simulink model "ITACG_3D_salvo_simulation"  (R2023b)
settings: Solver=ode4  StartTime=0.0  StopTime=28  FixedStep=1/10  RelTol=1e-3
libraries: simulink_extras x40, simulink x4
(part 1 of 2)
settings Model: NumberOfSteps=10  PacingRate=5  Creator=Administrator  LastModifiedBy=Administrator
settings DebuggingCC: UnderSpecifiedDimensionMsg=warning

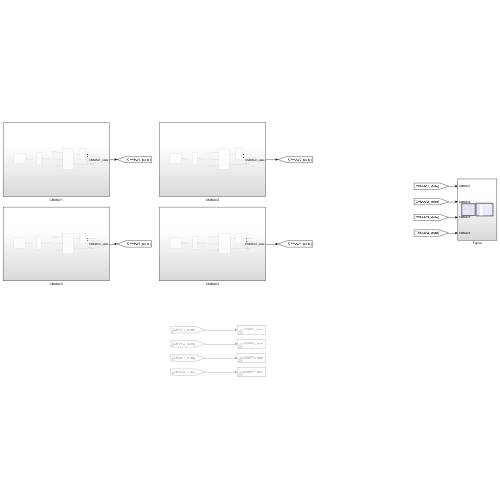
[thumbnail: Simulink's stored preview of the top-level diagram]
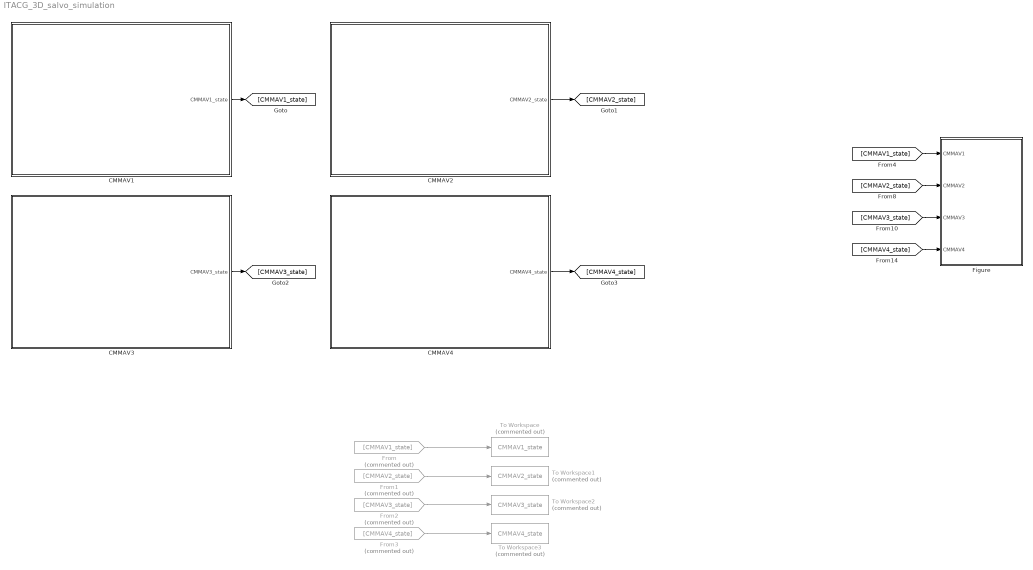
== system ITACG_3D_salvo_simulation ==
  CMMAV1 : Subsystem
  CMMAV2 : Subsystem
  CMMAV3 : Subsystem
  CMMAV4 : Subsystem
  Figure : Subsystem
  From : From  Commented=on  GotoTag=CMMAV1_state
  From1 : From  Commented=on  GotoTag=CMMAV2_state
  From2 : From  Commented=on  GotoTag=CMMAV3_state
  From3 : From  Commented=on  GotoTag=CMMAV4_state
  To Workspace : ToWorkspace  Commented=on  VariableName=CMMAV1_state  SaveFormat=Timeseries  SampleTime=-1
  To Workspace1 : ToWorkspace  Commented=on  VariableName=CMMAV2_state  SaveFormat=Timeseries  SampleTime=-1
  To Workspace2 : ToWorkspace  Commented=on  VariableName=CMMAV3_state  SaveFormat=Timeseries  SampleTime=-1
  To Workspace3 : ToWorkspace  Commented=on  VariableName=CMMAV4_state  SaveFormat=Timeseries  SampleTime=-1
  wires:
  CMMAV1/1(CMMAV1_state) -> [CMMAV1_state]
  CMMAV2/1(CMMAV2_state) -> [CMMAV2_state]
  CMMAV3/1(CMMAV3_state) -> [CMMAV3_state]
  CMMAV4/1(CMMAV4_state) -> [CMMAV4_state]
  From/1 -> To Workspace/1
  From1/1 -> To Workspace1/1
  From2/1 -> To Workspace2/1
  From3/1 -> To Workspace3/1
  [CMMAV2_state] -> Figure/2(CMMAV2)
  [CMMAV1_state] -> Figure/1(CMMAV1)
  [CMMAV3_state] -> Figure/3(CMMAV3)
  [CMMAV4_state] -> Figure/4(CMMAV4)

== system ITACG_3D_salvo_simulation/CMMAV1 ==
  Guidance : Subsystem
  Mux : Mux  Inputs=2
  Parameter init : Subsystem
  Point Mass Model : Subsystem
  Target : Subsystem  TreatAsAtomicUnit=on
  To File : ToFile  Filename=ITACG_CMMAV1.mat
  CMMAV1_state : Outport
  wires:
  [Parameter] -> Guidance/3(Parameter)
  [Taregt_info] -> Guidance/2(Target_info)
  [CMMAV1_state] -> Guidance/1(CMMAV1_state)
  Guidance/1(CMMAV1_input) -> Point Mass Model/1(CMMAV1_input)
  Parameter init/1(Parameter) -> [Parameter]
  Point Mass Model/1(CMMAV1_state) -> [CMMAV1_state], Mux/1, CMMAV1_state/1
  Target/1(Target_info) -> [Taregt_info]
  Mux/1 -> To File/1
  Guidance/2(sigma) -> Mux/2

== system ITACG_3D_salvo_simulation/CMMAV2 ==
  Guidance : Subsystem
  Mux : Mux  Inputs=2
  Parameter init : Subsystem
  Point Mass Model : Subsystem
  Target : Subsystem  TreatAsAtomicUnit=on
  To File : ToFile  Filename=ITACG_CMMAV2.mat
  CMMAV2_state : Outport
  wires:
  [Parameter] -> Guidance/3(Parameter)
  [Taregt_info] -> Guidance/2(Target_info)
  [CMMAV1_state] -> Guidance/1(CMMAV1_state)
  Guidance/1(CMMAV1_input) -> Point Mass Model/1(CMMAV1_input)
  Parameter init/1(Parameter) -> [Parameter]
  Target/1(Target_info) -> [Taregt_info]
  Point Mass Model/1(CMMAV1_state) -> CMMAV2_state/1, [CMMAV1_state], Mux/1
  Guidance/2(sigma) -> Mux/2
  Mux/1 -> To File/1

== system ITACG_3D_salvo_simulation/CMMAV3 ==
  Guidance : Subsystem
  Mux : Mux  Inputs=2
  Parameter init : Subsystem
  Point Mass Model : Subsystem
  Target : Subsystem  TreatAsAtomicUnit=on
  To File : ToFile  Filename=ITACG_CMMAV3.mat
  CMMAV3_state : Outport
  wires:
  [Parameter] -> Guidance/3(Parameter)
  [Taregt_info] -> Guidance/2(Target_info)
  [CMMAV1_state] -> Guidance/1(CMMAV1_state)
  Guidance/1(CMMAV1_input) -> Point Mass Model/1(CMMAV1_input)
  Parameter init/1(Parameter) -> [Parameter]
  Target/1(Target_info) -> [Taregt_info]
  Point Mass Model/1(CMMAV1_state) -> Mux/1, [CMMAV1_state], CMMAV3_state/1
  Guidance/2(sigma) -> Mux/2
  Mux/1 -> To File/1

== system ITACG_3D_salvo_simulation/CMMAV4 ==
  Guidance : Subsystem
  Mux : Mux  Inputs=2
  Parameter init : Subsystem
  Point Mass Model : Subsystem
  Target : Subsystem  TreatAsAtomicUnit=on
  To File : ToFile  Filename=ITACG_CMMAV4.mat
  CMMAV4_state : Outport
  wires:
  [Parameter] -> Guidance/3(Parameter)
  [Taregt_info] -> Guidance/2(Target_info)
  [CMMAV1_state] -> Guidance/1(CMMAV1_state)
  Guidance/1(CMMAV1_input) -> Point Mass Model/1(CMMAV1_input)
  Parameter init/1(Parameter) -> [Parameter]
  Target/1(Target_info) -> [Taregt_info]
  Point Mass Model/1(CMMAV1_state) -> Mux/1, [CMMAV1_state], CMMAV4_state/1
  Guidance/2(sigma) -> Mux/2
  Mux/1 -> To File/1

== system ITACG_3D_salvo_simulation/Figure ==
  note: Figure
  note: Input parameter
  CMMAV1 : Inport
  CMMAV2 : Inport  Port=2
  CMMAV3 : Inport  Port=3
  CMMAV4 : Inport  Port=4
  Bus Selector{,1..3} (4 alike) : BusSelector  OutputSignals=Pos_M_m
  Demux{,1..3} (4 alike) : Demux  Outputs=3
  MATLAB Function : MATLAB Function  TreatAsAtomicUnit=on
  wires:
  Demux/2 -> [CMMAV1_y]
  Demux/1 -> [CMMAV1_x]
  Demux/3 -> [CMMAV1_z]
  [CMMAV1] -> Demux/1
  CMMAV1/1 -> Bus Selector/1
  CMMAV2/1 -> Bus Selector1/1
  CMMAV3/1 -> Bus Selector2/1
  CMMAV4/1 -> Bus Selector3/1
  Bus Selector/1 -> [CMMAV1]  "<Pos_M_m>"
  Bus Selector1/1 -> [CMMAV2]  "<Pos_M_m>"
  Bus Selector2/1 -> [CMMAV3]  "<Pos_M_m>"
  Bus Selector3/1 -> [CMMAV4]  "<Pos_M_m>"
  Demux1/1 -> [CMMAV2_x]
  Demux1/3 -> [CMMAV2_z]
  Demux1/2 -> [CMMAV2_y]
  [CMMAV2] -> Demux1/1
  Demux2/2 -> [CMMAV3_y]
  Demux2/1 -> [CMMAV3_x]
  Demux2/3 -> [CMMAV3_z]
  [CMMAV3] -> Demux2/1
  Demux3/2 -> [CMMAV4_y]
  Demux3/1 -> [CMMAV4_x]
  Demux3/3 -> [CMMAV4_z]
  [CMMAV4] -> Demux3/1
  [CMMAV1_x] -> MATLAB Function/1(CMMAV1_x)
  [CMMAV1_y] -> MATLAB Function/2(CMMAV1_y)
  [CMMAV1_z] -> MATLAB Function/3(CMMAV1_z)
  [CMMAV2_x] -> MATLAB Function/4(CMMAV2_x)
  [CMMAV2_y] -> MATLAB Function/5(CMMAV2_y)
  [CMMAV2_z] -> MATLAB Function/6(CMMAV2_z)
  [CMMAV3_x] -> MATLAB Function/7(CMMAV3_x)
  [CMMAV3_y] -> MATLAB Function/8(CMMAV3_y)
  [CMMAV3_z] -> MATLAB Function/9(CMMAV3_z)
  [CMMAV4_x] -> MATLAB Function/10(CMMAV4_x)
  [CMMAV4_y] -> MATLAB Function/11(CMMAV4_y)
  [CMMAV4_z] -> MATLAB Function/12(CMMAV4_z)

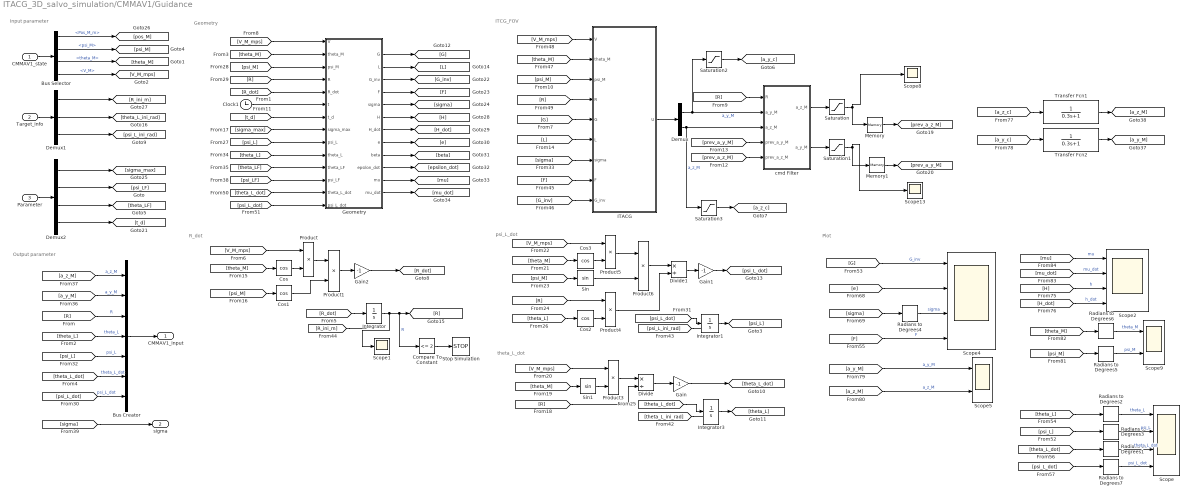
== system ITACG_3D_salvo_simulation/CMMAV1/Guidance ==
  note: Input parameter
  note: ITCG_FOV
  note: R_dot
  note: psi_L_dot
  note: theta_L_dot
  note: Output parameter
  note: Geometry
  note: Plot
  CMMAV1_state : Inport
  Target_info : Inport  Port=2
  Parameter : Inport  Port=3
  Bus Creator : BusCreator  Inputs=7
  Bus Selector : BusSelector  OutputSignals=Pos_M_m,psi_M,theta_M,V_M
  Clock1 : Clock
  Compare To Constant : simulink/Logic and Bit Operations/Compare To Constant  relop=<=  const=2  OutDataTypeStr=boolean
  Cos{,1..3} (4 alike) : Trigonometry  Operator=cos
  Demux : Demux  Outputs=2
  Demux1 : Demux  Outputs=3
  Demux2 : Demux
  Divide : Product  Inputs=*/
  Divide1 : Product  Inputs=*/
  Gain : Gain  Gain=-1
  Gain1 : Gain  Gain=-1
  Gain2 : Gain  Gain=-1
  Geometry : MATLAB Function  TreatAsAtomicUnit=on
  ITACG : MATLAB Function  TreatAsAtomicUnit=on
  Integrator : Integrator  InitialCondition=700
  Integrator1 : Integrator  InitialCondition=30*pi/180
  Integrator3 : Integrator  InitialCondition=-30*pi/180
  Memory : Memory
  Memory1 : Memory
  Product{,1,3..6} (6 alike) : Product
  Radians to Degrees{1..7} (7 alike) : simulink_extras/Transformations/Radians to Degrees
  Saturation{,1..3} (4 alike) : Saturate  UpperLimit=100  LowerLimit=-100
  Scope : Scope  NumInputPorts=4
  Scope1 : Scope
  Scope13 : Scope
  Scope2 : Scope  NumInputPorts=4
  Scope4 : Scope  NumInputPorts=4
  Scope5 : Scope  NumInputPorts=2
  Scope8 : Scope
  Scope9 : Scope  NumInputPorts=2
  Sin : Trigonometry
  Sin1 : Trigonometry
  Stop Simulation : Stop
  Transfer Fcn1 : TransferFcn  Denominator=[0.3 1]  ParameterTunability=Optimized
  Transfer Fcn2 : TransferFcn  Denominator=[0.3 1]  ParameterTunability=Optimized
  cmd Filter : MATLAB Function  TreatAsAtomicUnit=on
  CMMAV1_input : Outport
  sigma : Outport  Port=2
  wires:
  Product1/1 -> Gain2/1
  Gain2/1 -> [R_dot]
  [theta_L] -> Cos2/1
  [theta_L_dot] -> Integrator3/1
  Gain/1 -> [theta_L_dot]
  Product5/1 -> Product6/1
  Divide1/1 -> Gain1/1
  [V_M_mps] -> Product3/1
  [V_M_mps] -> Product5/1
  [theta_M] -> Sin1/1
  [R] -> Divide/2
  [theta_M] -> Cos3/1
  Divide/1 -> Gain/1
  [theta_M] -> Cos/1
  [R] -> Product4/1
  Product4/1 -> Divide1/2
  Integrator3/1 -> [theta_L]
  [psi_L_dot] -> Integrator1/1
  Sin1/1 -> Product3/2
  Product3/1 -> Divide/1
  [psi_M] -> Cos1/1
  Cos/1 -> Product/2
  Integrator1/1 -> [psi_L]
  Product6/1 -> Divide1/1
  [psi_M] -> Sin/1
  Compare To Constant/1 -> Stop Simulation/1
  [V_M_mps] -> Product/1
  Cos3/1 -> Product5/2
  Sin/1 -> Product6/2
  Integrator/1 -> Scope1/1, [R], Compare To Constant/1  "R"
  Product/1 -> Product1/1
  Cos2/1 -> Product4/2
  Cos1/1 -> Product1/2
  Gain1/1 -> [psi_L_dot]
  [R_dot] -> Integrator/1
  CMMAV1_state/1 -> Bus Selector/1
  Target_info/1 -> Demux1/1
  Demux2/1 -> [sigma_max]
  Parameter/1 -> Demux2/1
  Bus Selector/1 -> [pos_M]  "<Pos_M_m>"
  Bus Selector/4 -> [V_M_mps]  "<V_M>"
  Demux1/2 -> [theta_L_ini_rad]
  Demux1/3 -> [psi_L_ini_rad]
  Demux1/1 -> [R_ini_m]
  [psi_L] -> Bus Creator/5  "psi_L"
  [theta_L] -> Bus Creator/4  "theta_L"
  Bus Creator/1 -> CMMAV1_input/1
  [a_y_M] -> Bus Creator/2  "a_y_M"
  [R] -> Bus Creator/3  "R"
  [a_z_M] -> Bus Creator/1  "a_z_M"
  [theta_L_ini_rad] -> ?
  [psi_L_ini_rad] -> ?
  [R_ini_m] -> ?
  Bus Selector/2 -> [psi_M]  "<psi_M>"
  Bus Selector/3 -> [theta_M]  "<theta_M>"
  [psi_M] -> Geometry/3(psi_M)
  [V_M_mps] -> Geometry/1(V)
  [theta_M] -> Geometry/2(theta_M)
  [R] -> Geometry/4(R)
  Demux2/2 -> [psi_LF]
  Demux2/3 -> [theta_LF]
  Demux2/4 -> [t_d]
  Saturation2/1 -> [a_y_c]
  Saturation3/1 -> [a_z_c]
  cmd Filter/1(a_z_M) -> Saturation/1
  Memory/1 -> [prev_a_z_M]
  Transfer Fcn2/1 -> [a_y_M]
  Transfer Fcn1/1 -> [a_z_M]
  cmd Filter/2(a_y_M) -> Saturation1/1
  Saturation1/1 -> Scope13/1, Memory1/1
  Saturation/1 -> Scope8/1, Memory/1
  Demux/2 -> cmd Filter/3("a_z_M "), Saturation3/1  "a_z_M"
  [prev_a_y_M] -> cmd Filter/4(prev_a_y_M)
  [prev_a_z_M] -> cmd Filter/5(prev_a_z_M)
  [a_z_c] -> Transfer Fcn1/1
  Demux/1 -> cmd Filter/2("a_y_M "), Saturation2/1  "a_y_M"
  Memory1/1 -> [prev_a_y_M]
  [a_y_c] -> Transfer Fcn2/1
  [R] -> cmd Filter/1(R)
  ITACG/1(U) -> Demux/1
  [theta_LF] -> Geometry/11(theta_LF)
  [psi_LF] -> Geometry/12(psi_LF)
  [theta_L_dot] -> Geometry/13(theta_L_dot)
  [R_dot] -> Geometry/5(R_dot)
  [t_d] -> Geometry/7(t_d)
  [sigma_max] -> Geometry/8(sigma_max)
  [psi_L] -> Geometry/9(psi_L)
  [theta_L] -> Geometry/10(theta_L)
  [psi_L_dot] -> Geometry/14(psi_L_dot)
  Clock1/1 -> Geometry/6(t)
  Geometry/1(G) -> [G]
  Geometry/2(L) -> [L]
  Geometry/3(G_inv) -> [G_inv]
  Geometry/4(F) -> [F]
  Geometry/5(sigma) -> [sigma]
  Geometry/6(H) -> [H]
  Geometry/7(H_dot) -> [H_dot]
  Geometry/8(e) -> [e]
  Geometry/9(beta) -> [beta]
  Geometry/10(epsilon_dot) -> [epsilon_dot]
  Geometry/11(mu) -> [mu]
  Geometry/12(mu_dot) -> [mu_dot]
  [V_M_mps] -> ITACG/1(V)
  [theta_M] -> ITACG/2(theta_M)
  [psi_M] -> ITACG/3(psi_M)
  [G] -> ITACG/5(G)
  [L] -> ITACG/6(L)
  [sigma] -> ITACG/7(sigma)
  [F] -> ITACG/8(F)
  [G_inv] -> ITACG/9(G_inv)
  [R] -> ITACG/4(R)
  Radians to Degrees6/1 -> Scope9/1  "theta_M"
  Radians to Degrees7/1 -> Scope/4  "psi_L_dot"
  [psi_M] -> Radians to Degrees5/1
  [theta_L_dot] -> Radians to Degrees1/1
  Radians to Degrees3/1 -> Scope/2  "psi_L"
  [theta_L] -> Radians to Degrees2/1
  Radians to Degrees4/1 -> Scope4/3  "sigma"
  Radians to Degrees2/1 -> Scope/1  "theta_L"
  Radians to Degrees5/1 -> Scope9/2  "psi_M"
  [H] -> Scope2/3  "h"
  [psi_L] -> Radians to Degrees3/1
  [mu] -> Scope2/1  "mu"
  [mu_dot] -> Scope2/2  "mu_dot"
  Radians to Degrees1/1 -> Scope/3  "theta_L_dot"
  [sigma] -> Radians to Degrees4/1
  [a_y_M] -> Scope5/1  "a_y_M"
  [a_z_M] -> Scope5/2  "a_z_M"
  [G] -> Scope4/1  "G_inv"
  [theta_M] -> Radians to Degrees6/1
  [psi_L_dot] -> Radians to Degrees7/1
  [F] -> Scope4/4  "F"
  [H_dot] -> Scope2/4  "h_dot"
  [e] -> Scope4/2
  [theta_L_dot] -> Bus Creator/6  "theta_L_dot"
  [psi_L_dot] -> Bus Creator/7  "psi_L_dot"
  [sigma] -> sigma/1

== system ITACG_3D_salvo_simulation/CMMAV1/Parameter init ==
  Constant : Constant  Value=45
  Constant1 : Constant  Value=0
  Constant2 : Constant  Value=-60
  Constant3 : Constant  Value=28
  Degrees to Radians : simulink_extras/Transformations/Degrees to Radians
  Degrees to Radians1 : simulink_extras/Transformations/Degrees to Radians
  Degrees to Radians2 : simulink_extras/Transformations/Degrees to Radians
  Mux : Mux
  Parameter : Outport
  wires:
  Mux/1 -> Parameter/1
  Constant3/1 -> Mux/4  "t_d"
  Constant2/1 -> Degrees to Radians2/1
  Constant1/1 -> Degrees to Radians1/1
  Constant/1 -> Degrees to Radians/1
  Degrees to Radians2/1 -> Mux/3  "theta_LF"
  Degrees to Radians1/1 -> Mux/2  "psi_LF"
  Degrees to Radians/1 -> Mux/1  "sigma_max"

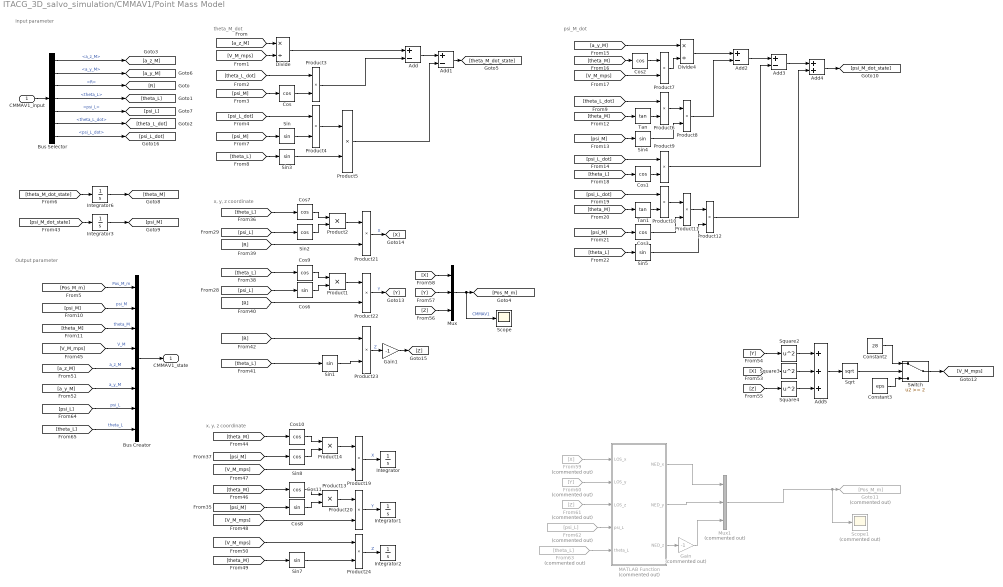
== system ITACG_3D_salvo_simulation/CMMAV1/Point Mass Model ==
  note: Input parameter
  note: x, y, z coordinate
  note: Output parameter
  note: x, y, z coordinate
  note: theta_M_dot
  note: psi_M_dot
  CMMAV1_input : Inport
  Add{,1..3} (4 alike) : Sum  Inputs=+-
  Add4 : Sum
  Add5 : Sum  Inputs=+++
  Bus Creator : BusCreator  Inputs=8
  Bus Selector : BusSelector  OutputSignals=a_z_M,a_y_M,R,theta_L,psi_L,theta_L_dot,psi_L_dot
  Constant2 : Constant  Value=28
  Constant3 : Constant  Value=eps
  Cos{,1..3,7,9..11} (8 alike) : Trigonometry  Operator=cos
  Cos6 : Trigonometry
  Cos8 : Trigonometry
  Divide : Product  Inputs=*/
  Divide4 : Product  Inputs=*/
  From59 : From  Commented=on  GotoTag=X
  From60 : From  Commented=on  GotoTag=Y
  From61 : From  Commented=on  GotoTag=Z
  From62 : From  Commented=on  GotoTag=psi_L
  From63 : From  Commented=on  GotoTag=theta_L
  Gain : Gain  Commented=on  Gain=-1
  Gain1 : Gain  Gain=-1
  Goto11 : Goto  Commented=on  GotoTag=Pos_M_m
  Integrator : Integrator
  Integrator1 : Integrator
  Integrator2 : Integrator
  Integrator3 : Integrator  InitialCondition=10*pi/180
  Integrator6 : Integrator  InitialCondition=10*pi/180
  MATLAB Function : MATLAB Function  Commented=on  TreatAsAtomicUnit=on
  Mux : Mux  Inputs=3
  Mux1 : Mux  Commented=on  Inputs=3
  Product{1..14,19..24} (20 alike) : Product
  Scope : Scope
  Scope1 : Scope  Commented=on
  Sin{,1,3..5,7} (6 alike) : Trigonometry
  Sin2 : Trigonometry  Operator=cos
  Sin8 : Trigonometry  Operator=cos
  Sqrt : Sqrt
  Square2 : Math  Operator=square
  Square3 : Math  Operator=square
  Square4 : Math  Operator=square
  Switch : Switch  Threshold=2  SaturateOnIntegerOverflow=off  InputSameDT=off
  Tan : Trigonometry  Operator=tan
  Tan1 : Trigonometry  Operator=tan
  CMMAV1_state : Outport
  wires:
  [psi_M] -> Bus Creator/2  "psi_M"
  [psi_M_dot_state] -> Integrator3/1
  [theta_L] -> Cos9/1
  [V_M_mps] -> Bus Creator/4  "V_M"
  Cos6/1 -> Product1/2
  Bus Selector/2 -> [a_y_M]  "<a_y_M>"
  Integrator6/1 -> [theta_M]
  [psi_L] -> Cos6/1
  Bus Selector/5 -> [psi_L]  "<psi_L>"
  Product21/1 -> [X]  "X"
  Product1/1 -> Product22/1
  Integrator3/1 -> [psi_M]
  Sin2/1 -> Product2/2
  Bus Selector/1 -> [a_z_M]  "<a_z_M>"
  Mux/1 -> [Pos_M_m], Scope/1  "CMMAV1"
  Bus Selector/3 -> [R]  "<R>"
  [theta_M] -> Bus Creator/3  "theta_M"
  [psi_L] -> Sin2/1
  Product2/1 -> Product21/1
  Cos9/1 -> Product1/1
  [theta_L] -> Cos7/1
  Cos7/1 -> Product2/1
  [theta_M_dot_state] -> Integrator6/1
  Product22/1 -> [Y]  "Y"
  [V_M_mps] -> Product24/1
  Sin7/1 -> Product24/2
  [V_M_mps] -> Product20/2
  [theta_M] -> Cos11/1
  [psi_M] -> Sin8/1
  [theta_M] -> Sin7/1
  Sin8/1 -> Product14/2
  Product14/1 -> Product19/1
  Product19/1 -> Integrator/1  "X"
  Product13/1 -> Product20/1
  Product24/1 -> Integrator2/1  "Z"
  [psi_M] -> Cos8/1
  [V_M_mps] -> Product19/2
  [theta_M] -> Cos10/1
  Cos11/1 -> Product13/1
  Cos8/1 -> Product13/2
  Product20/1 -> Integrator1/1  "Y"
  Cos10/1 -> Product14/1
  [R] -> Product21/2
  [R] -> Product22/2
  [R] -> Product23/1
  Sin1/1 -> Product23/2
  [theta_L] -> Sin1/1
  CMMAV1_input/1 -> Bus Selector/1
  [Pos_M_m] -> Bus Creator/1  "Pos_M_m"
  Bus Creator/1 -> CMMAV1_state/1
  Bus Selector/4 -> [theta_L]  "<theta_L>"
  [a_z_M] -> Bus Creator/5  "a_z_M"
  [a_y_M] -> Bus Creator/6  "a_y_M"
  Constant3/1 -> Switch/3
  Switch/1 -> [V_M_mps]
  Sqrt/1 -> Switch/2
  Add5/1 -> Sqrt/1
  Square2/1 -> Add5/1
  [Y] -> Square2/1
  Constant2/1 -> Switch/1
  [X] -> Square3/1
  Square3/1 -> Add5/2
  Product23/1 -> Gain1/1  "Z"
  [Z] -> Square4/1
  [X] -> Mux/1
  [Y] -> Mux/2
  [Z] -> Mux/3
  Square4/1 -> Add5/3
  From59/1 -> MATLAB Function/1(LOS_x)
  From60/1 -> MATLAB Function/2(LOS_y)
  From61/1 -> MATLAB Function/3(LOS_z)
  From62/1 -> MATLAB Function/4(psi_L)
  From63/1 -> MATLAB Function/5(theta_L)
  MATLAB Function/2(NED_y) -> Mux1/2
  MATLAB Function/1(NED_x) -> Mux1/1
  MATLAB Function/3(NED_z) -> Gain/1
  Gain/1 -> Mux1/3
  Mux1/1 -> Scope1/1, Goto11/1
  [psi_L] -> Bus Creator/7  "psi_L"
  [theta_L] -> Bus Creator/8  "theta_L"
  Product5/1 -> Add1/2
  Add/1 -> Add1/1
  Product4/1 -> Product5/1
  [a_z_M] -> Divide/1
  Divide/1 -> Add/1
  [V_M_mps] -> Divide/2
  Sin3/1 -> Product5/2
  Sin/1 -> Product4/2
  [psi_L_dot] -> Product4/1
  [psi_M] -> Cos/1
  Cos/1 -> Product3/2
  Add1/1 -> [theta_M_dot_state]
  Product3/1 -> Add/2
  [psi_M] -> Sin/1
  [theta_L] -> Sin3/1
  [theta_L_dot] -> Product3/1
  Product8/1 -> Add2/2
  [a_y_M] -> Divide4/1
  Product7/1 -> Divide4/2
  Divide4/1 -> Add2/1
  [V_M_mps] -> Product7/2
  Product6/1 -> Product8/1
  Product10/1 -> Product11/1
  Tan1/1 -> Product10/2
  [theta_L] -> Cos1/1
  Product12/1 -> Add4/2
  [theta_L] -> Sin5/1
  Product11/1 -> Product12/1
  [theta_L_dot] -> Product6/1
  Sin5/1 -> Product12/2
  Cos3/1 -> Product11/2
  [psi_M] -> Cos3/1
  Product9/1 -> Add3/2
  Add4/1 -> [psi_M_dot_state]
  [psi_L_dot] -> Product10/1
  [theta_M] -> Tan1/1
  Cos1/1 -> Product9/2
  [theta_M] -> Cos2/1
  Sin4/1 -> Product8/2
  [psi_M] -> Sin4/1
  [theta_M] -> Tan/1
  Tan/1 -> Product6/2
  [psi_L_dot] -> Product9/1
  Cos2/1 -> Product7/1
  Add2/1 -> Add3/1
  Add3/1 -> Add4/1
  Gain1/1 -> [Z]
  Bus Selector/6 -> [theta_L_dot]  "<theta_L_dot>"
  Bus Selector/7 -> [psi_L_dot]  "<psi_L_dot>"

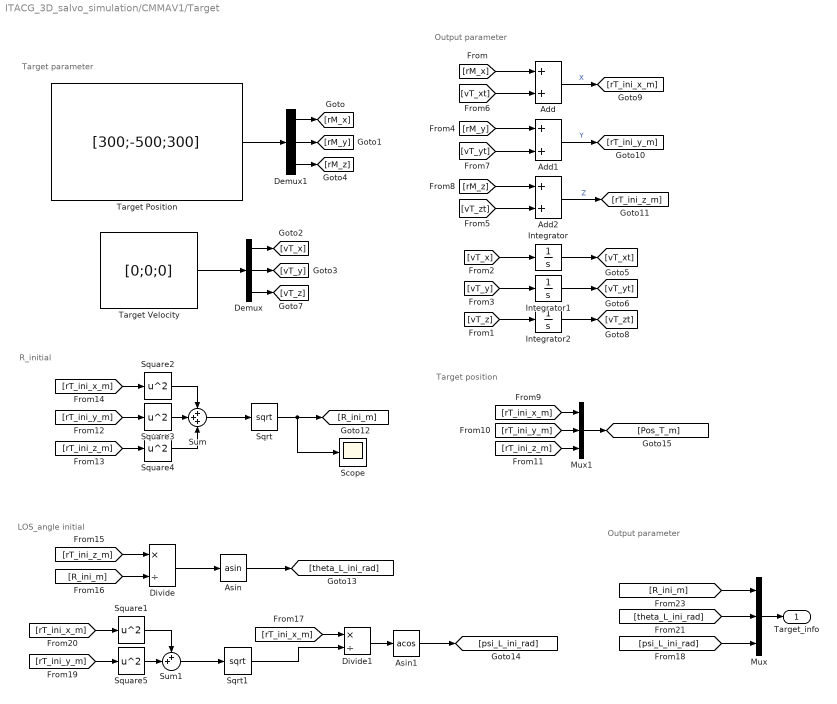
== system ITACG_3D_salvo_simulation/CMMAV1/Target ==
  note: LOS_angle initial
  note: Target position
  note: Target parameter
  note: Output parameter
  note: R_initial
  note: Output parameter
  Add : Sum
  Add1 : Sum
  Add2 : Sum
  Asin : Trigonometry  Operator=asin
  Asin1 : Trigonometry  Operator=acos
  Demux : Demux  Outputs=3
  Demux1 : Demux  Outputs=3
  Divide : Product  Inputs=*/
  Divide1 : Product  Inputs=*/
  Integrator : Integrator
  Integrator1 : Integrator
  Integrator2 : Integrator
  Mux : Mux  Inputs=3
  Mux1 : Mux  Inputs=3
  Scope : Scope
  Sqrt : Sqrt
  Sqrt1 : Sqrt
  Square{1..5} (5 alike) : Math  Operator=square
  Sum : Sum  Inputs=+++
  Sum1 : Sum  Inputs=++|
  Target Position : Constant  Value=[300;-500;300]  VectorParams1D=off
  Target Velocity : Constant  Value=[0;0;0]  VectorParams1D=off
  Target_info : Outport
  wires:
  [psi_L_ini_rad] -> Mux/3
  Asin/1 -> [theta_L_ini_rad]
  [rT_ini_z_m] -> Mux1/3
  [rM_z] -> Add2/1
  Demux/3 -> [vT_z]
  [vT_z] -> Integrator2/1
  Demux/2 -> [vT_y]
  [rT_ini_x_m] -> Mux1/1
  Add1/1 -> [rT_ini_y_m]  "Y"
  Square2/1 -> Sum/1
  [vT_x] -> Integrator/1
  Mux1/1 -> [Pos_T_m]
  Square3/1 -> Sum/2
  Add2/1 -> [rT_ini_z_m]  "Z"
  Integrator/1 -> [vT_xt]
  Sum/1 -> Sqrt/1
  Demux1/3 -> [rM_z]
  [rT_ini_y_m] -> Mux1/2
  Integrator1/1 -> [vT_yt]
  Demux/1 -> [vT_x]
  Demux1/1 -> [rM_x]
  Target Velocity/1 -> Demux/1
  Demux1/2 -> [rM_y]
  Add/1 -> [rT_ini_x_m]  "X"
  [vT_yt] -> Add1/2
  Divide1/1 -> Asin1/1
  [rM_x] -> Add/1
  [vT_zt] -> Add2/2
  Sum1/1 -> Sqrt1/1
  [rT_ini_x_m] -> Square1/1
  Square1/1 -> Sum1/1
  Square5/1 -> Sum1/2
  [rT_ini_y_m] -> Square5/1
  [vT_y] -> Integrator1/1
  [rM_y] -> Add1/1
  [rT_ini_z_m] -> Divide/1
  [R_ini_m] -> Mux/1
  Sqrt/1 -> Scope/1, [R_ini_m]
  [R_ini_m] -> Divide/2
  [rT_ini_z_m] -> Square4/1
  Sqrt1/1 -> Divide1/2
  [vT_xt] -> Add/2
  Divide/1 -> Asin/1
  Integrator2/1 -> [vT_zt]
  Square4/1 -> Sum/3
  [rT_ini_x_m] -> Divide1/1
  [theta_L_ini_rad] -> Mux/2
  Asin1/1 -> [psi_L_ini_rad]
  Mux/1 -> Target_info/1
  Target Position/1 -> Demux1/1
  [rT_ini_y_m] -> Square3/1
  [rT_ini_x_m] -> Square2/1

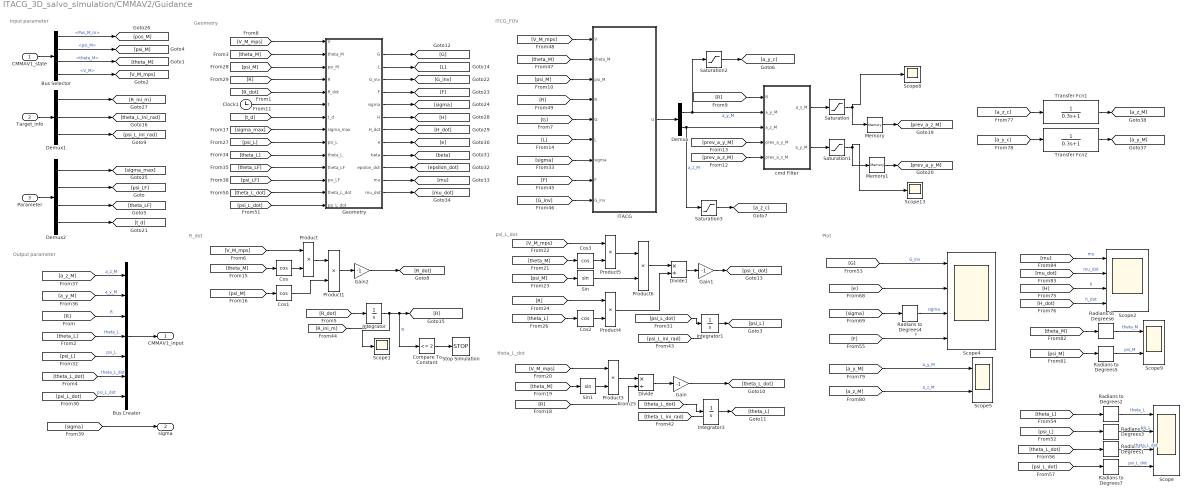
== system ITACG_3D_salvo_simulation/CMMAV2/Guidance ==
  note: Input parameter
  note: ITCG_FOV
  note: R_dot
  note: psi_L_dot
  note: theta_L_dot
  note: Output parameter
  note: Geometry
  note: Plot
  CMMAV1_state : Inport
  Target_info : Inport  Port=2
  Parameter : Inport  Port=3
  Bus Creator : BusCreator  Inputs=7
  Bus Selector : BusSelector  OutputSignals=Pos_M_m,psi_M,theta_M,V_M
  Clock1 : Clock
  Compare To Constant : simulink/Logic and Bit Operations/Compare To Constant  relop=<=  const=2  OutDataTypeStr=boolean
  Cos{,1..3} (4 alike) : Trigonometry  Operator=cos
  Demux : Demux  Outputs=2
  Demux1 : Demux  Outputs=3
  Demux2 : Demux
  Divide : Product  Inputs=*/
  Divide1 : Product  Inputs=*/
  Gain : Gain  Gain=-1
  Gain1 : Gain  Gain=-1
  Gain2 : Gain  Gain=-1
  Geometry : MATLAB Function  TreatAsAtomicUnit=on
  ITACG : MATLAB Function  TreatAsAtomicUnit=on
  Integrator : Integrator  InitialCondition=700
  Integrator1 : Integrator  InitialCondition=-30*pi/180
  Integrator3 : Integrator  InitialCondition=-30*pi/180
  Memory : Memory
  Memory1 : Memory
  Product{,1,3..6} (6 alike) : Product
  Radians to Degrees{1..7} (7 alike) : simulink_extras/Transformations/Radians to Degrees
  Saturation{,1..3} (4 alike) : Saturate  UpperLimit=100  LowerLimit=-100
  Scope : Scope  NumInputPorts=4
  Scope1 : Scope
  Scope13 : Scope
  Scope2 : Scope  NumInputPorts=4
  Scope4 : Scope  NumInputPorts=4
  Scope5 : Scope  NumInputPorts=2
  Scope8 : Scope
  Scope9 : Scope  NumInputPorts=2
  Sin : Trigonometry
  Sin1 : Trigonometry
  Stop Simulation : Stop
  Transfer Fcn1 : TransferFcn  Denominator=[0.3 1]  ParameterTunability=Optimized
  Transfer Fcn2 : TransferFcn  Denominator=[0.3 1]  ParameterTunability=Optimized
  cmd Filter : MATLAB Function  TreatAsAtomicUnit=on
  CMMAV1_input : Outport
  sigma : Outport  Port=2
  wires:
  Product1/1 -> Gain2/1
  Gain2/1 -> [R_dot]
  [theta_L] -> Cos2/1
  [theta_L_dot] -> Integrator3/1
  Gain/1 -> [theta_L_dot]
  Product5/1 -> Product6/1
  Divide1/1 -> Gain1/1
  [V_M_mps] -> Product3/1
  [V_M_mps] -> Product5/1
  [theta_M] -> Sin1/1
  [R] -> Divide/2
  [theta_M] -> Cos3/1
  Divide/1 -> Gain/1
  [theta_M] -> Cos/1
  [R] -> Product4/1
  Product4/1 -> Divide1/2
  Integrator3/1 -> [theta_L]
  [psi_L_dot] -> Integrator1/1
  Sin1/1 -> Product3/2
  Product3/1 -> Divide/1
  [psi_M] -> Cos1/1
  Cos/1 -> Product/2
  Integrator1/1 -> [psi_L]
  Product6/1 -> Divide1/1
  [psi_M] -> Sin/1
  Compare To Constant/1 -> Stop Simulation/1
  [V_M_mps] -> Product/1
  Cos3/1 -> Product5/2
  Sin/1 -> Product6/2
  Integrator/1 -> Scope1/1, [R], Compare To Constant/1  "R"
  Product/1 -> Product1/1
  Cos2/1 -> Product4/2
  Cos1/1 -> Product1/2
  Gain1/1 -> [psi_L_dot]
  [R_dot] -> Integrator/1
  CMMAV1_state/1 -> Bus Selector/1
  Target_info/1 -> Demux1/1
  Demux2/1 -> [sigma_max]
  Parameter/1 -> Demux2/1
  Bus Selector/1 -> [pos_M]  "<Pos_M_m>"
  Bus Selector/4 -> [V_M_mps]  "<V_M>"
  Demux1/2 -> [theta_L_ini_rad]
  Demux1/3 -> [psi_L_ini_rad]
  Demux1/1 -> [R_ini_m]
  [psi_L] -> Bus Creator/5  "psi_L"
  [theta_L] -> Bus Creator/4  "theta_L"
  Bus Creator/1 -> CMMAV1_input/1
  [a_y_M] -> Bus Creator/2  "a_y_M"
  [R] -> Bus Creator/3  "R"
  [a_z_M] -> Bus Creator/1  "a_z_M"
  [theta_L_ini_rad] -> ?
  [psi_L_ini_rad] -> ?
  [R_ini_m] -> ?
  Bus Selector/2 -> [psi_M]  "<psi_M>"
  Bus Selector/3 -> [theta_M]  "<theta_M>"
  [psi_M] -> Geometry/3(psi_M)
  [V_M_mps] -> Geometry/1(V)
  [theta_M] -> Geometry/2(theta_M)
  [R] -> Geometry/4(R)
  Demux2/2 -> [psi_LF]
  Demux2/3 -> [theta_LF]
  Demux2/4 -> [t_d]
  Saturation2/1 -> [a_y_c]
  Saturation3/1 -> [a_z_c]
  cmd Filter/1(a_z_M) -> Saturation/1
  Memory/1 -> [prev_a_z_M]
  Transfer Fcn2/1 -> [a_y_M]
  Transfer Fcn1/1 -> [a_z_M]
  cmd Filter/2(a_y_M) -> Saturation1/1
  Saturation1/1 -> Scope13/1, Memory1/1
  Saturation/1 -> Scope8/1, Memory/1
  Demux/2 -> cmd Filter/3("a_z_M "), Saturation3/1  "a_z_M"
  [prev_a_y_M] -> cmd Filter/4(prev_a_y_M)
  [prev_a_z_M] -> cmd Filter/5(prev_a_z_M)
  [a_z_c] -> Transfer Fcn1/1
  Demux/1 -> cmd Filter/2("a_y_M "), Saturation2/1  "a_y_M"
  Memory1/1 -> [prev_a_y_M]
  [a_y_c] -> Transfer Fcn2/1
  [R] -> cmd Filter/1(R)
  ITACG/1(U) -> Demux/1
  [theta_LF] -> Geometry/11(theta_LF)
  [psi_LF] -> Geometry/12(psi_LF)
  [theta_L_dot] -> Geometry/13(theta_L_dot)
  [R_dot] -> Geometry/5(R_dot)
  [t_d] -> Geometry/7(t_d)
  [sigma_max] -> Geometry/8(sigma_max)
  [psi_L] -> Geometry/9(psi_L)
  [theta_L] -> Geometry/10(theta_L)
  [psi_L_dot] -> Geometry/14(psi_L_dot)
  Clock1/1 -> Geometry/6(t)
  Geometry/1(G) -> [G]
  Geometry/2(L) -> [L]
  Geometry/3(G_inv) -> [G_inv]
  Geometry/4(F) -> [F]
  Geometry/5(sigma) -> [sigma]
  Geometry/6(H) -> [H]
  Geometry/7(H_dot) -> [H_dot]
  Geometry/8(e) -> [e]
  Geometry/9(beta) -> [beta]
  Geometry/10(epsilon_dot) -> [epsilon_dot]
  Geometry/11(mu) -> [mu]
  Geometry/12(mu_dot) -> [mu_dot]
  [V_M_mps] -> ITACG/1(V)
  [theta_M] -> ITACG/2(theta_M)
  [psi_M] -> ITACG/3(psi_M)
  [G] -> ITACG/5(G)
  [L] -> ITACG/6(L)
  [sigma] -> ITACG/7(sigma)
  [F] -> ITACG/8(F)
  [G_inv] -> ITACG/9(G_inv)
  [R] -> ITACG/4(R)
  Radians to Degrees6/1 -> Scope9/1  "theta_M"
  Radians to Degrees7/1 -> Scope/4  "psi_L_dot"
  [psi_M] -> Radians to Degrees5/1
  [theta_L_dot] -> Radians to Degrees1/1
  Radians to Degrees3/1 -> Scope/2  "psi_L"
  [theta_L] -> Radians to Degrees2/1
  Radians to Degrees4/1 -> Scope4/3  "sigma"
  Radians to Degrees2/1 -> Scope/1  "theta_L"
  Radians to Degrees5/1 -> Scope9/2  "psi_M"
  [H] -> Scope2/3  "h"
  [psi_L] -> Radians to Degrees3/1
  [mu] -> Scope2/1  "mu"
  [mu_dot] -> Scope2/2  "mu_dot"
  Radians to Degrees1/1 -> Scope/3  "theta_L_dot"
  [sigma] -> Radians to Degrees4/1
  [a_y_M] -> Scope5/1  "a_y_M"
  [a_z_M] -> Scope5/2  "a_z_M"
  [G] -> Scope4/1  "G_inv"
  [theta_M] -> Radians to Degrees6/1
  [psi_L_dot] -> Radians to Degrees7/1
  [F] -> Scope4/4  "F"
  [H_dot] -> Scope2/4  "h_dot"
  [e] -> Scope4/2
  [theta_L_dot] -> Bus Creator/6  "theta_L_dot"
  [psi_L_dot] -> Bus Creator/7  "psi_L_dot"
  [sigma] -> sigma/1

== system ITACG_3D_salvo_simulation/CMMAV2/Parameter init ==
  Constant : Constant  Value=45
  Constant1 : Constant  Value=0
  Constant2 : Constant  Value=-70
  Constant3 : Constant  Value=28
  Degrees to Radians : simulink_extras/Transformations/Degrees to Radians
  Degrees to Radians1 : simulink_extras/Transformations/Degrees to Radians
  Degrees to Radians2 : simulink_extras/Transformations/Degrees to Radians
  Mux : Mux
  Parameter : Outport
  wires:
  Mux/1 -> Parameter/1
  Constant3/1 -> Mux/4  "t_d"
  Constant2/1 -> Degrees to Radians2/1
  Constant1/1 -> Degrees to Radians1/1
  Constant/1 -> Degrees to Radians/1
  Degrees to Radians2/1 -> Mux/3  "theta_LF"
  Degrees to Radians1/1 -> Mux/2  "psi_LF"
  Degrees to Radians/1 -> Mux/1  "sigma_max"

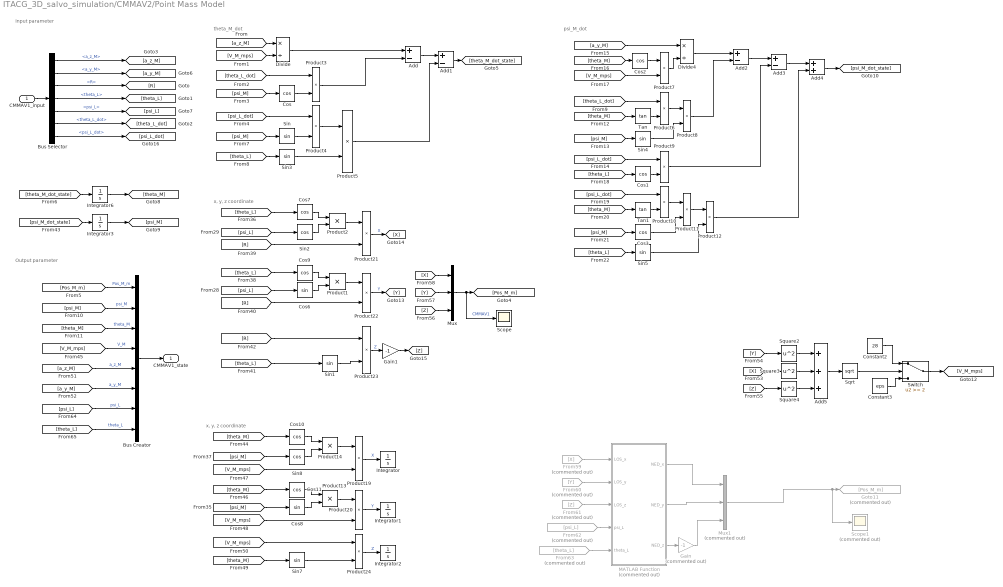
== system ITACG_3D_salvo_simulation/CMMAV2/Point Mass Model ==
  note: Input parameter
  note: x, y, z coordinate
  note: Output parameter
  note: x, y, z coordinate
  note: theta_M_dot
  note: psi_M_dot
  CMMAV1_input : Inport
  Add{,1..3} (4 alike) : Sum  Inputs=+-
  Add4 : Sum
  Add5 : Sum  Inputs=+++
  Bus Creator : BusCreator  Inputs=8
  Bus Selector : BusSelector  OutputSignals=a_z_M,a_y_M,R,theta_L,psi_L,theta_L_dot,psi_L_dot
  Constant2 : Constant  Value=28
  Constant3 : Constant  Value=eps
  Cos{,1..3,7,9..11} (8 alike) : Trigonometry  Operator=cos
  Cos6 : Trigonometry
  Cos8 : Trigonometry
  Divide : Product  Inputs=*/
  Divide4 : Product  Inputs=*/
  From59 : From  Commented=on  GotoTag=X
  From60 : From  Commented=on  GotoTag=Y
  From61 : From  Commented=on  GotoTag=Z
  From62 : From  Commented=on  GotoTag=psi_L
  From63 : From  Commented=on  GotoTag=theta_L
  Gain : Gain  Commented=on  Gain=-1
  Gain1 : Gain  Gain=-1
  Goto11 : Goto  Commented=on  GotoTag=Pos_M_m
  Integrator : Integrator
  Integrator1 : Integrator
  Integrator2 : Integrator
  Integrator3 : Integrator  InitialCondition=10*pi/180
  Integrator6 : Integrator  InitialCondition=10*pi/180
  MATLAB Function : MATLAB Function  Commented=on  TreatAsAtomicUnit=on
  Mux : Mux  Inputs=3
  Mux1 : Mux  Commented=on  Inputs=3
  Product{1..14,19..24} (20 alike) : Product
  Scope : Scope
  Scope1 : Scope  Commented=on
  Sin{,1,3..5,7} (6 alike) : Trigonometry
  Sin2 : Trigonometry  Operator=cos
  Sin8 : Trigonometry  Operator=cos
  Sqrt : Sqrt
  Square2 : Math  Operator=square
  Square3 : Math  Operator=square
  Square4 : Math  Operator=square
  Switch : Switch  Threshold=2  SaturateOnIntegerOverflow=off  InputSameDT=off
  Tan : Trigonometry  Operator=tan
  Tan1 : Trigonometry  Operator=tan
  CMMAV1_state : Outport
  wires:
  [psi_M] -> Bus Creator/2  "psi_M"
  [psi_M_dot_state] -> Integrator3/1
  [theta_L] -> Cos9/1
  [V_M_mps] -> Bus Creator/4  "V_M"
  Cos6/1 -> Product1/2
  Bus Selector/2 -> [a_y_M]  "<a_y_M>"
  Integrator6/1 -> [theta_M]
  [psi_L] -> Cos6/1
  Bus Selector/5 -> [psi_L]  "<psi_L>"
  Product21/1 -> [X]  "X"
  Product1/1 -> Product22/1
  Integrator3/1 -> [psi_M]
  Sin2/1 -> Product2/2
  Bus Selector/1 -> [a_z_M]  "<a_z_M>"
  Mux/1 -> [Pos_M_m], Scope/1  "CMMAV1"
  Bus Selector/3 -> [R]  "<R>"
  [theta_M] -> Bus Creator/3  "theta_M"
  [psi_L] -> Sin2/1
  Product2/1 -> Product21/1
  Cos9/1 -> Product1/1
  [theta_L] -> Cos7/1
  Cos7/1 -> Product2/1
  [theta_M_dot_state] -> Integrator6/1
  Product22/1 -> [Y]  "Y"
  [V_M_mps] -> Product24/1
  Sin7/1 -> Product24/2
  [V_M_mps] -> Product20/2
  [theta_M] -> Cos11/1
  [psi_M] -> Sin8/1
  [theta_M] -> Sin7/1
  Sin8/1 -> Product14/2
  Product14/1 -> Product19/1
  Product19/1 -> Integrator/1  "X"
  Product13/1 -> Product20/1
  Product24/1 -> Integrator2/1  "Z"
  [psi_M] -> Cos8/1
  [V_M_mps] -> Product19/2
  [theta_M] -> Cos10/1
  Cos11/1 -> Product13/1
  Cos8/1 -> Product13/2
  Product20/1 -> Integrator1/1  "Y"
  Cos10/1 -> Product14/1
  [R] -> Product21/2
  [R] -> Product22/2
  [R] -> Product23/1
  Sin1/1 -> Product23/2
  [theta_L] -> Sin1/1
  CMMAV1_input/1 -> Bus Selector/1
  [Pos_M_m] -> Bus Creator/1  "Pos_M_m"
  Bus Creator/1 -> CMMAV1_state/1
  Bus Selector/4 -> [theta_L]  "<theta_L>"
  [a_z_M] -> Bus Creator/5  "a_z_M"
  [a_y_M] -> Bus Creator/6  "a_y_M"
  Constant3/1 -> Switch/3
  Switch/1 -> [V_M_mps]
  Sqrt/1 -> Switch/2
  Add5/1 -> Sqrt/1
  Square2/1 -> Add5/1
  [Y] -> Square2/1
  Constant2/1 -> Switch/1
  [X] -> Square3/1
  Square3/1 -> Add5/2
  Product23/1 -> Gain1/1  "Z"
  [Z] -> Square4/1
  [X] -> Mux/1
  [Y] -> Mux/2
  [Z] -> Mux/3
  Square4/1 -> Add5/3
  From59/1 -> MATLAB Function/1(LOS_x)
  From60/1 -> MATLAB Function/2(LOS_y)
  From61/1 -> MATLAB Function/3(LOS_z)
  From62/1 -> MATLAB Function/4(psi_L)
  From63/1 -> MATLAB Function/5(theta_L)
  MATLAB Function/2(NED_y) -> Mux1/2
  MATLAB Function/1(NED_x) -> Mux1/1
  MATLAB Function/3(NED_z) -> Gain/1
  Gain/1 -> Mux1/3
  Mux1/1 -> Scope1/1, Goto11/1
  [psi_L] -> Bus Creator/7  "psi_L"
  [theta_L] -> Bus Creator/8  "theta_L"
  Product5/1 -> Add1/2
  Add/1 -> Add1/1
  Product4/1 -> Product5/1
  [a_z_M] -> Divide/1
  Divide/1 -> Add/1
  [V_M_mps] -> Divide/2
  Sin3/1 -> Product5/2
  Sin/1 -> Product4/2
  [psi_L_dot] -> Product4/1
  [psi_M] -> Cos/1
  Cos/1 -> Product3/2
  Add1/1 -> [theta_M_dot_state]
  Product3/1 -> Add/2
  [psi_M] -> Sin/1
  [theta_L] -> Sin3/1
  [theta_L_dot] -> Product3/1
  Product8/1 -> Add2/2
  [a_y_M] -> Divide4/1
  Product7/1 -> Divide4/2
  Divide4/1 -> Add2/1
  [V_M_mps] -> Product7/2
  Product6/1 -> Product8/1
  Product10/1 -> Product11/1
  Tan1/1 -> Product10/2
  [theta_L] -> Cos1/1
  Product12/1 -> Add4/2
  [theta_L] -> Sin5/1
  Product11/1 -> Product12/1
  [theta_L_dot] -> Product6/1
  Sin5/1 -> Product12/2
  Cos3/1 -> Product11/2
  [psi_M] -> Cos3/1
  Product9/1 -> Add3/2
  Add4/1 -> [psi_M_dot_state]
  [psi_L_dot] -> Product10/1
  [theta_M] -> Tan1/1
  Cos1/1 -> Product9/2
  [theta_M] -> Cos2/1
  Sin4/1 -> Product8/2
  [psi_M] -> Sin4/1
  [theta_M] -> Tan/1
  Tan/1 -> Product6/2
  [psi_L_dot] -> Product9/1
  Cos2/1 -> Product7/1
  Add2/1 -> Add3/1
  Add3/1 -> Add4/1
  Gain1/1 -> [Z]
  Bus Selector/6 -> [theta_L_dot]  "<theta_L_dot>"
  Bus Selector/7 -> [psi_L_dot]  "<psi_L_dot>"

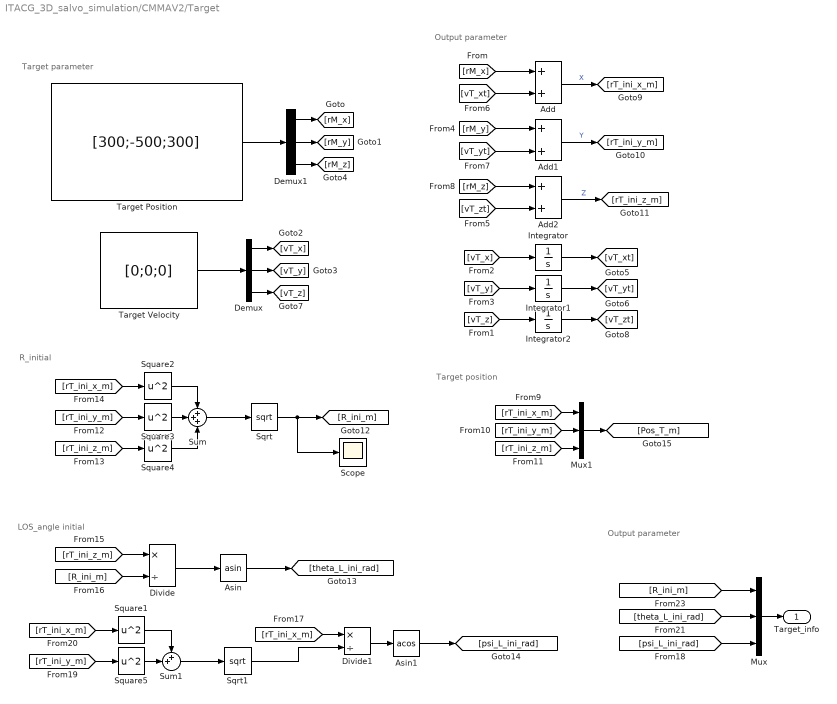
== system ITACG_3D_salvo_simulation/CMMAV2/Target ==
  note: LOS_angle initial
  note: Target position
  note: Target parameter
  note: Output parameter
  note: R_initial
  note: Output parameter
  Add : Sum
  Add1 : Sum
  Add2 : Sum
  Asin : Trigonometry  Operator=asin
  Asin1 : Trigonometry  Operator=acos
  Demux : Demux  Outputs=3
  Demux1 : Demux  Outputs=3
  Divide : Product  Inputs=*/
  Divide1 : Product  Inputs=*/
  Integrator : Integrator
  Integrator1 : Integrator
  Integrator2 : Integrator
  Mux : Mux  Inputs=3
  Mux1 : Mux  Inputs=3
  Scope : Scope
  Sqrt : Sqrt
  Sqrt1 : Sqrt
  Square{1..5} (5 alike) : Math  Operator=square
  Sum : Sum  Inputs=+++
  Sum1 : Sum  Inputs=++|
  Target Position : Constant  Value=[300;-500;300]  VectorParams1D=off
  Target Velocity : Constant  Value=[0;0;0]  VectorParams1D=off
  Target_info : Outport
  wires:
  [psi_L_ini_rad] -> Mux/3
  Asin/1 -> [theta_L_ini_rad]
  [rT_ini_z_m] -> Mux1/3
  [rM_z] -> Add2/1
  Demux/3 -> [vT_z]
  [vT_z] -> Integrator2/1
  Demux/2 -> [vT_y]
  [rT_ini_x_m] -> Mux1/1
  Add1/1 -> [rT_ini_y_m]  "Y"
  Square2/1 -> Sum/1
  [vT_x] -> Integrator/1
  Mux1/1 -> [Pos_T_m]
  Square3/1 -> Sum/2
  Add2/1 -> [rT_ini_z_m]  "Z"
  Integrator/1 -> [vT_xt]
  Sum/1 -> Sqrt/1
  Demux1/3 -> [rM_z]
  [rT_ini_y_m] -> Mux1/2
  Integrator1/1 -> [vT_yt]
  Demux/1 -> [vT_x]
  Demux1/1 -> [rM_x]
  Target Velocity/1 -> Demux/1
  Demux1/2 -> [rM_y]
  Add/1 -> [rT_ini_x_m]  "X"
  [vT_yt] -> Add1/2
  Divide1/1 -> Asin1/1
  [rM_x] -> Add/1
  [vT_zt] -> Add2/2
  Sum1/1 -> Sqrt1/1
  [rT_ini_x_m] -> Square1/1
  Square1/1 -> Sum1/1
  Square5/1 -> Sum1/2
  [rT_ini_y_m] -> Square5/1
  [vT_y] -> Integrator1/1
  [rM_y] -> Add1/1
  [rT_ini_z_m] -> Divide/1
  [R_ini_m] -> Mux/1
  Sqrt/1 -> Scope/1, [R_ini_m]
  [R_ini_m] -> Divide/2
  [rT_ini_z_m] -> Square4/1
  Sqrt1/1 -> Divide1/2
  [vT_xt] -> Add/2
  Divide/1 -> Asin/1
  Integrator2/1 -> [vT_zt]
  Square4/1 -> Sum/3
  [rT_ini_x_m] -> Divide1/1
  [theta_L_ini_rad] -> Mux/2
  Asin1/1 -> [psi_L_ini_rad]
  Mux/1 -> Target_info/1
  Target Position/1 -> Demux1/1
  [rT_ini_y_m] -> Square3/1
  [rT_ini_x_m] -> Square2/1

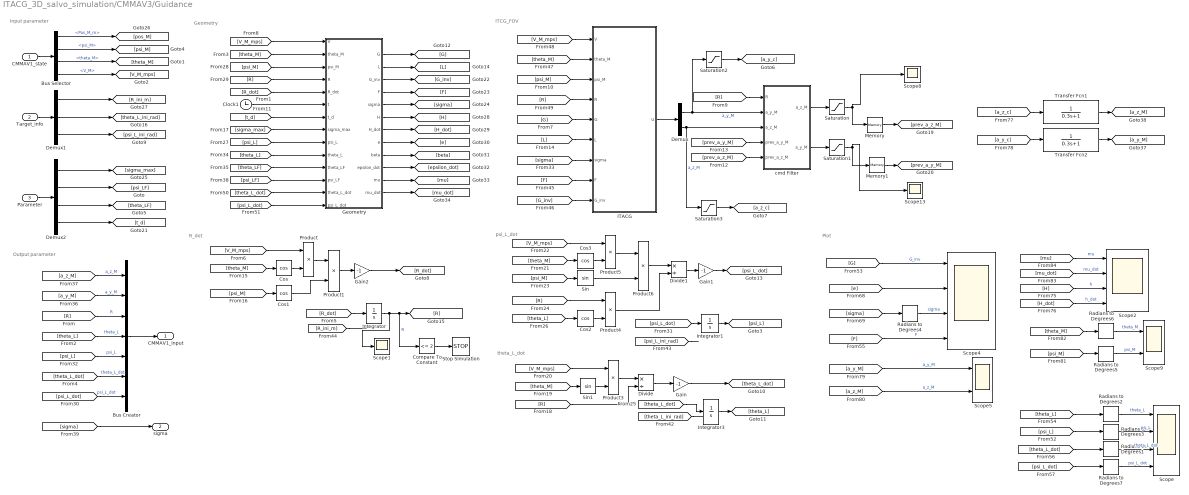
== system ITACG_3D_salvo_simulation/CMMAV3/Guidance ==
  note: Input parameter
  note: ITCG_FOV
  note: R_dot
  note: psi_L_dot
  note: theta_L_dot
  note: Output parameter
  note: Geometry
  note: Plot
  CMMAV1_state : Inport
  Target_info : Inport  Port=2
  Parameter : Inport  Port=3
  Bus Creator : BusCreator  Inputs=7
  Bus Selector : BusSelector  OutputSignals=Pos_M_m,psi_M,theta_M,V_M
  Clock1 : Clock
  Compare To Constant : simulink/Logic and Bit Operations/Compare To Constant  relop=<=  const=2  OutDataTypeStr=boolean
  Cos{,1..3} (4 alike) : Trigonometry  Operator=cos
  Demux : Demux  Outputs=2
  Demux1 : Demux  Outputs=3
  Demux2 : Demux
  Divide : Product  Inputs=*/
  Divide1 : Product  Inputs=*/
  Gain : Gain  Gain=-1
  Gain1 : Gain  Gain=-1
  Gain2 : Gain  Gain=-1
  Geometry : MATLAB Function  TreatAsAtomicUnit=on
  ITACG : MATLAB Function  TreatAsAtomicUnit=on
  Integrator : Integrator  InitialCondition=700
  Integrator1 : Integrator  InitialCondition=20*pi/180
  Integrator3 : Integrator  InitialCondition=-10*pi/180
  Memory : Memory
  Memory1 : Memory
  Product{,1,3..6} (6 alike) : Product
  Radians to Degrees{1..7} (7 alike) : simulink_extras/Transformations/Radians to Degrees
  Saturation{,1..3} (4 alike) : Saturate  UpperLimit=100  LowerLimit=-100
  Scope : Scope  NumInputPorts=4
  Scope1 : Scope
  Scope13 : Scope
  Scope2 : Scope  NumInputPorts=4
  Scope4 : Scope  NumInputPorts=4
  Scope5 : Scope  NumInputPorts=2
  Scope8 : Scope
  Scope9 : Scope  NumInputPorts=2
  Sin : Trigonometry
  Sin1 : Trigonometry
  Stop Simulation : Stop
  Transfer Fcn1 : TransferFcn  Denominator=[0.3 1]  ParameterTunability=Optimized
  Transfer Fcn2 : TransferFcn  Denominator=[0.3 1]  ParameterTunability=Optimized
  cmd Filter : MATLAB Function  TreatAsAtomicUnit=on
  CMMAV1_input : Outport
  sigma : Outport  Port=2
  wires:
  Product1/1 -> Gain2/1
  Gain2/1 -> [R_dot]
  [theta_L] -> Cos2/1
  [theta_L_dot] -> Integrator3/1
  Gain/1 -> [theta_L_dot]
  Product5/1 -> Product6/1
  Divide1/1 -> Gain1/1
  [V_M_mps] -> Product3/1
  [V_M_mps] -> Product5/1
  [theta_M] -> Sin1/1
  [R] -> Divide/2
  [theta_M] -> Cos3/1
  Divide/1 -> Gain/1
  [theta_M] -> Cos/1
  [R] -> Product4/1
  Product4/1 -> Divide1/2
  Integrator3/1 -> [theta_L]
  [psi_L_dot] -> Integrator1/1
  Sin1/1 -> Product3/2
  Product3/1 -> Divide/1
  [psi_M] -> Cos1/1
  Cos/1 -> Product/2
  Integrator1/1 -> [psi_L]
  Product6/1 -> Divide1/1
  [psi_M] -> Sin/1
  Compare To Constant/1 -> Stop Simulation/1
  [V_M_mps] -> Product/1
  Cos3/1 -> Product5/2
  Sin/1 -> Product6/2
  Integrator/1 -> Scope1/1, [R], Compare To Constant/1  "R"
  Product/1 -> Product1/1
  Cos2/1 -> Product4/2
  Cos1/1 -> Product1/2
  Gain1/1 -> [psi_L_dot]
  [R_dot] -> Integrator/1
  CMMAV1_state/1 -> Bus Selector/1
  Target_info/1 -> Demux1/1
  Demux2/1 -> [sigma_max]
  Parameter/1 -> Demux2/1
  Bus Selector/1 -> [pos_M]  "<Pos_M_m>"
  Bus Selector/4 -> [V_M_mps]  "<V_M>"
  Demux1/2 -> [theta_L_ini_rad]
  Demux1/3 -> [psi_L_ini_rad]
  Demux1/1 -> [R_ini_m]
  [psi_L] -> Bus Creator/5  "psi_L"
  [theta_L] -> Bus Creator/4  "theta_L"
  Bus Creator/1 -> CMMAV1_input/1
  [a_y_M] -> Bus Creator/2  "a_y_M"
  [R] -> Bus Creator/3  "R"
  [a_z_M] -> Bus Creator/1  "a_z_M"
  [theta_L_ini_rad] -> ?
  [psi_L_ini_rad] -> ?
  [R_ini_m] -> ?
  Bus Selector/2 -> [psi_M]  "<psi_M>"
  Bus Selector/3 -> [theta_M]  "<theta_M>"
  [psi_M] -> Geometry/3(psi_M)
  [V_M_mps] -> Geometry/1(V)
  [theta_M] -> Geometry/2(theta_M)
  [R] -> Geometry/4(R)
  Demux2/2 -> [psi_LF]
  Demux2/3 -> [theta_LF]
  Demux2/4 -> [t_d]
  Saturation2/1 -> [a_y_c]
  Saturation3/1 -> [a_z_c]
  cmd Filter/1(a_z_M) -> Saturation/1
  Memory/1 -> [prev_a_z_M]
  Transfer Fcn2/1 -> [a_y_M]
  Transfer Fcn1/1 -> [a_z_M]
  cmd Filter/2(a_y_M) -> Saturation1/1
  Saturation1/1 -> Scope13/1, Memory1/1
  Saturation/1 -> Scope8/1, Memory/1
  Demux/2 -> cmd Filter/3("a_z_M "), Saturation3/1  "a_z_M"
  [prev_a_y_M] -> cmd Filter/4(prev_a_y_M)
  [prev_a_z_M] -> cmd Filter/5(prev_a_z_M)
  [a_z_c] -> Transfer Fcn1/1
  Demux/1 -> cmd Filter/2("a_y_M "), Saturation2/1  "a_y_M"
  Memory1/1 -> [prev_a_y_M]
  [a_y_c] -> Transfer Fcn2/1
  [R] -> cmd Filter/1(R)
  ITACG/1(U) -> Demux/1
  [theta_LF] -> Geometry/11(theta_LF)
  [psi_LF] -> Geometry/12(psi_LF)
  [theta_L_dot] -> Geometry/13(theta_L_dot)
  [R_dot] -> Geometry/5(R_dot)
  [t_d] -> Geometry/7(t_d)
  [sigma_max] -> Geometry/8(sigma_max)
  [psi_L] -> Geometry/9(psi_L)
  [theta_L] -> Geometry/10(theta_L)
  [psi_L_dot] -> Geometry/14(psi_L_dot)
  Clock1/1 -> Geometry/6(t)
  Geometry/1(G) -> [G]
  Geometry/2(L) -> [L]
  Geometry/3(G_inv) -> [G_inv]
  Geometry/4(F) -> [F]
  Geometry/5(sigma) -> [sigma]
  Geometry/6(H) -> [H]
  Geometry/7(H_dot) -> [H_dot]
  Geometry/8(e) -> [e]
  Geometry/9(beta) -> [beta]
  Geometry/10(epsilon_dot) -> [epsilon_dot]
  Geometry/11(mu) -> [mu]
  Geometry/12(mu_dot) -> [mu_dot]
  [V_M_mps] -> ITACG/1(V)
  [theta_M] -> ITACG/2(theta_M)
  [psi_M] -> ITACG/3(psi_M)
  [G] -> ITACG/5(G)
  [L] -> ITACG/6(L)
  [sigma] -> ITACG/7(sigma)
  [F] -> ITACG/8(F)
  [G_inv] -> ITACG/9(G_inv)
  [R] -> ITACG/4(R)
  Radians to Degrees6/1 -> Scope9/1  "theta_M"
  Radians to Degrees7/1 -> Scope/4  "psi_L_dot"
  [psi_M] -> Radians to Degrees5/1
  [theta_L_dot] -> Radians to Degrees1/1
  Radians to Degrees3/1 -> Scope/2  "psi_L"
  [theta_L] -> Radians to Degrees2/1
  Radians to Degrees4/1 -> Scope4/3  "sigma"
  Radians to Degrees2/1 -> Scope/1  "theta_L"
  Radians to Degrees5/1 -> Scope9/2  "psi_M"
  [H] -> Scope2/3  "h"
  [psi_L] -> Radians to Degrees3/1
  [mu] -> Scope2/1  "mu"
  [mu_dot] -> Scope2/2  "mu_dot"
  Radians to Degrees1/1 -> Scope/3  "theta_L_dot"
  [sigma] -> Radians to Degrees4/1
  [a_y_M] -> Scope5/1  "a_y_M"
  [a_z_M] -> Scope5/2  "a_z_M"
  [G] -> Scope4/1  "G_inv"
  [theta_M] -> Radians to Degrees6/1
  [psi_L_dot] -> Radians to Degrees7/1
  [F] -> Scope4/4  "F"
  [H_dot] -> Scope2/4  "h_dot"
  [e] -> Scope4/2
  [theta_L_dot] -> Bus Creator/6  "theta_L_dot"
  [psi_L_dot] -> Bus Creator/7  "psi_L_dot"
  [sigma] -> sigma/1

== system ITACG_3D_salvo_simulation/CMMAV3/Parameter init ==
  Constant : Constant  Value=45
  Constant1 : Constant  Value=00
  Constant2 : Constant  Value=-50
  Constant3 : Constant  Value=28
  Degrees to Radians : simulink_extras/Transformations/Degrees to Radians
  Degrees to Radians1 : simulink_extras/Transformations/Degrees to Radians
  Degrees to Radians2 : simulink_extras/Transformations/Degrees to Radians
  Mux : Mux
  Parameter : Outport
  wires:
  Mux/1 -> Parameter/1
  Constant3/1 -> Mux/4  "t_d"
  Constant2/1 -> Degrees to Radians2/1
  Constant1/1 -> Degrees to Radians1/1
  Constant/1 -> Degrees to Radians/1
  Degrees to Radians2/1 -> Mux/3  "theta_LF"
  Degrees to Radians1/1 -> Mux/2  "psi_LF"
  Degrees to Radians/1 -> Mux/1  "sigma_max"

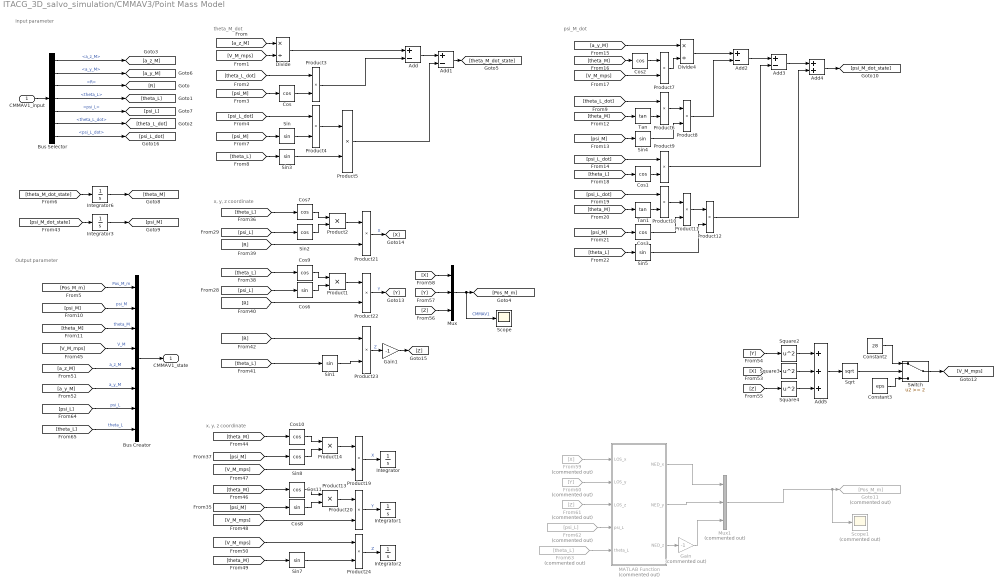
== system ITACG_3D_salvo_simulation/CMMAV3/Point Mass Model ==
  note: Input parameter
  note: x, y, z coordinate
  note: Output parameter
  note: x, y, z coordinate
  note: theta_M_dot
  note: psi_M_dot
  CMMAV1_input : Inport
  Add{,1..3} (4 alike) : Sum  Inputs=+-
  Add4 : Sum
  Add5 : Sum  Inputs=+++
  Bus Creator : BusCreator  Inputs=8
  Bus Selector : BusSelector  OutputSignals=a_z_M,a_y_M,R,theta_L,psi_L,theta_L_dot,psi_L_dot
  Constant2 : Constant  Value=28
  Constant3 : Constant  Value=eps
  Cos{,1..3,7,9..11} (8 alike) : Trigonometry  Operator=cos
  Cos6 : Trigonometry
  Cos8 : Trigonometry
  Divide : Product  Inputs=*/
  Divide4 : Product  Inputs=*/
  From59 : From  Commented=on  GotoTag=X
  From60 : From  Commented=on  GotoTag=Y
  From61 : From  Commented=on  GotoTag=Z
  From62 : From  Commented=on  GotoTag=psi_L
  From63 : From  Commented=on  GotoTag=theta_L
  Gain : Gain  Commented=on  Gain=-1
  Gain1 : Gain  Gain=-1
  Goto11 : Goto  Commented=on  GotoTag=Pos_M_m
  Integrator : Integrator
  Integrator1 : Integrator
  Integrator2 : Integrator
  Integrator3 : Integrator  InitialCondition=30*pi/180
  Integrator6 : Integrator  InitialCondition=20*pi/180
  MATLAB Function : MATLAB Function  Commented=on  TreatAsAtomicUnit=on
  Mux : Mux  Inputs=3
  Mux1 : Mux  Commented=on  Inputs=3
  Product{1..14,19..24} (20 alike) : Product
  Scope : Scope
  Scope1 : Scope  Commented=on
  Sin{,1,3..5,7} (6 alike) : Trigonometry
  Sin2 : Trigonometry  Operator=cos
  Sin8 : Trigonometry  Operator=cos
  Sqrt : Sqrt
  Square2 : Math  Operator=square
  Square3 : Math  Operator=square
  Square4 : Math  Operator=square
  Switch : Switch  Threshold=2  SaturateOnIntegerOverflow=off  InputSameDT=off
  Tan : Trigonometry  Operator=tan
  Tan1 : Trigonometry  Operator=tan
  CMMAV1_state : Outport
  wires:
  [psi_M] -> Bus Creator/2  "psi_M"
  [psi_M_dot_state] -> Integrator3/1
  [theta_L] -> Cos9/1
  [V_M_mps] -> Bus Creator/4  "V_M"
  Cos6/1 -> Product1/2
  Bus Selector/2 -> [a_y_M]  "<a_y_M>"
  Integrator6/1 -> [theta_M]
  [psi_L] -> Cos6/1
  Bus Selector/5 -> [psi_L]  "<psi_L>"
  Product21/1 -> [X]  "X"
  Product1/1 -> Product22/1
  Integrator3/1 -> [psi_M]
  Sin2/1 -> Product2/2
  Bus Selector/1 -> [a_z_M]  "<a_z_M>"
  Mux/1 -> [Pos_M_m], Scope/1  "CMMAV1"
  Bus Selector/3 -> [R]  "<R>"
  [theta_M] -> Bus Creator/3  "theta_M"
  [psi_L] -> Sin2/1
  Product2/1 -> Product21/1
  Cos9/1 -> Product1/1
  [theta_L] -> Cos7/1
  Cos7/1 -> Product2/1
  [theta_M_dot_state] -> Integrator6/1
  Product22/1 -> [Y]  "Y"
  [V_M_mps] -> Product24/1
  Sin7/1 -> Product24/2
  [V_M_mps] -> Product20/2
  [theta_M] -> Cos11/1
  [psi_M] -> Sin8/1
  [theta_M] -> Sin7/1
  Sin8/1 -> Product14/2
  Product14/1 -> Product19/1
  Product19/1 -> Integrator/1  "X"
  Product13/1 -> Product20/1
  Product24/1 -> Integrator2/1  "Z"
  [psi_M] -> Cos8/1
  [V_M_mps] -> Product19/2
  [theta_M] -> Cos10/1
  Cos11/1 -> Product13/1
  Cos8/1 -> Product13/2
  Product20/1 -> Integrator1/1  "Y"
  Cos10/1 -> Product14/1
  [R] -> Product21/2
  [R] -> Product22/2
  [R] -> Product23/1
  Sin1/1 -> Product23/2
  [theta_L] -> Sin1/1
  CMMAV1_input/1 -> Bus Selector/1
  [Pos_M_m] -> Bus Creator/1  "Pos_M_m"
  Bus Creator/1 -> CMMAV1_state/1
  Bus Selector/4 -> [theta_L]  "<theta_L>"
  [a_z_M] -> Bus Creator/5  "a_z_M"
  [a_y_M] -> Bus Creator/6  "a_y_M"
  Constant3/1 -> Switch/3
  Switch/1 -> [V_M_mps]
  Sqrt/1 -> Switch/2
  Add5/1 -> Sqrt/1
  Square2/1 -> Add5/1
  [Y] -> Square2/1
  Constant2/1 -> Switch/1
  [X] -> Square3/1
  Square3/1 -> Add5/2
  Product23/1 -> Gain1/1  "Z"
  [Z] -> Square4/1
  [X] -> Mux/1
  [Y] -> Mux/2
  [Z] -> Mux/3
  Square4/1 -> Add5/3
  From59/1 -> MATLAB Function/1(LOS_x)
  From60/1 -> MATLAB Function/2(LOS_y)
  From61/1 -> MATLAB Function/3(LOS_z)
  From62/1 -> MATLAB Function/4(psi_L)
  From63/1 -> MATLAB Function/5(theta_L)
  MATLAB Function/2(NED_y) -> Mux1/2
  MATLAB Function/1(NED_x) -> Mux1/1
  MATLAB Function/3(NED_z) -> Gain/1
  Gain/1 -> Mux1/3
  Mux1/1 -> Scope1/1, Goto11/1
  [psi_L] -> Bus Creator/7  "psi_L"
  [theta_L] -> Bus Creator/8  "theta_L"
  Product5/1 -> Add1/2
  Add/1 -> Add1/1
  Product4/1 -> Product5/1
  [a_z_M] -> Divide/1
  Divide/1 -> Add/1
  [V_M_mps] -> Divide/2
  Sin3/1 -> Product5/2
  Sin/1 -> Product4/2
  [psi_L_dot] -> Product4/1
  [psi_M] -> Cos/1
  Cos/1 -> Product3/2
  Add1/1 -> [theta_M_dot_state]
  Product3/1 -> Add/2
  [psi_M] -> Sin/1
  [theta_L] -> Sin3/1
  [theta_L_dot] -> Product3/1
  Product8/1 -> Add2/2
  [a_y_M] -> Divide4/1
  Product7/1 -> Divide4/2
  Divide4/1 -> Add2/1
  [V_M_mps] -> Product7/2
  Product6/1 -> Product8/1
  Product10/1 -> Product11/1
  Tan1/1 -> Product10/2
  [theta_L] -> Cos1/1
  Product12/1 -> Add4/2
  [theta_L] -> Sin5/1
  Product11/1 -> Product12/1
  [theta_L_dot] -> Product6/1
  Sin5/1 -> Product12/2
  Cos3/1 -> Product11/2
  [psi_M] -> Cos3/1
  Product9/1 -> Add3/2
  Add4/1 -> [psi_M_dot_state]
  [psi_L_dot] -> Product10/1
  [theta_M] -> Tan1/1
  Cos1/1 -> Product9/2
  [theta_M] -> Cos2/1
  Sin4/1 -> Product8/2
  [psi_M] -> Sin4/1
  [theta_M] -> Tan/1
  Tan/1 -> Product6/2
  [psi_L_dot] -> Product9/1
  Cos2/1 -> Product7/1
  Add2/1 -> Add3/1
  Add3/1 -> Add4/1
  Gain1/1 -> [Z]
  Bus Selector/6 -> [theta_L_dot]  "<theta_L_dot>"
  Bus Selector/7 -> [psi_L_dot]  "<psi_L_dot>"

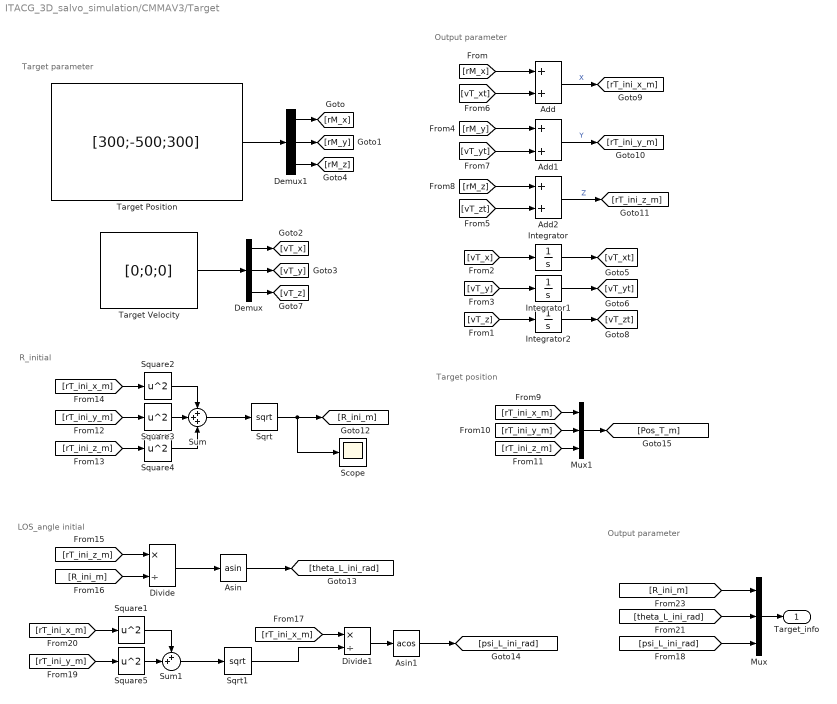
== system ITACG_3D_salvo_simulation/CMMAV3/Target ==
  note: LOS_angle initial
  note: Target position
  note: Target parameter
  note: Output parameter
  note: R_initial
  note: Output parameter
  Add : Sum
  Add1 : Sum
  Add2 : Sum
  Asin : Trigonometry  Operator=asin
  Asin1 : Trigonometry  Operator=acos
  Demux : Demux  Outputs=3
  Demux1 : Demux  Outputs=3
  Divide : Product  Inputs=*/
  Divide1 : Product  Inputs=*/
  Integrator : Integrator
  Integrator1 : Integrator
  Integrator2 : Integrator
  Mux : Mux  Inputs=3
  Mux1 : Mux  Inputs=3
  Scope : Scope
  Sqrt : Sqrt
  Sqrt1 : Sqrt
  Square{1..5} (5 alike) : Math  Operator=square
  Sum : Sum  Inputs=+++
  Sum1 : Sum  Inputs=++|
  Target Position : Constant  Value=[300;-500;300]  VectorParams1D=off
  Target Velocity : Constant  Value=[0;0;0]  VectorParams1D=off
  Target_info : Outport
  wires:
  [psi_L_ini_rad] -> Mux/3
  Asin/1 -> [theta_L_ini_rad]
  [rT_ini_z_m] -> Mux1/3
  [rM_z] -> Add2/1
  Demux/3 -> [vT_z]
  [vT_z] -> Integrator2/1
  Demux/2 -> [vT_y]
  [rT_ini_x_m] -> Mux1/1
  Add1/1 -> [rT_ini_y_m]  "Y"
  Square2/1 -> Sum/1
  [vT_x] -> Integrator/1
  Mux1/1 -> [Pos_T_m]
  Square3/1 -> Sum/2
  Add2/1 -> [rT_ini_z_m]  "Z"
  Integrator/1 -> [vT_xt]
  Sum/1 -> Sqrt/1
  Demux1/3 -> [rM_z]
  [rT_ini_y_m] -> Mux1/2
  Integrator1/1 -> [vT_yt]
  Demux/1 -> [vT_x]
  Demux1/1 -> [rM_x]
  Target Velocity/1 -> Demux/1
  Demux1/2 -> [rM_y]
  Add/1 -> [rT_ini_x_m]  "X"
  [vT_yt] -> Add1/2
  Divide1/1 -> Asin1/1
  [rM_x] -> Add/1
  [vT_zt] -> Add2/2
  Sum1/1 -> Sqrt1/1
  [rT_ini_x_m] -> Square1/1
  Square1/1 -> Sum1/1
  Square5/1 -> Sum1/2
  [rT_ini_y_m] -> Square5/1
  [vT_y] -> Integrator1/1
  [rM_y] -> Add1/1
  [rT_ini_z_m] -> Divide/1
  [R_ini_m] -> Mux/1
  Sqrt/1 -> Scope/1, [R_ini_m]
  [R_ini_m] -> Divide/2
  [rT_ini_z_m] -> Square4/1
  Sqrt1/1 -> Divide1/2
  [vT_xt] -> Add/2
  Divide/1 -> Asin/1
  Integrator2/1 -> [vT_zt]
  Square4/1 -> Sum/3
  [rT_ini_x_m] -> Divide1/1
  [theta_L_ini_rad] -> Mux/2
  Asin1/1 -> [psi_L_ini_rad]
  Mux/1 -> Target_info/1
  Target Position/1 -> Demux1/1
  [rT_ini_y_m] -> Square3/1
  [rT_ini_x_m] -> Square2/1
